simulink model "FKtest"  (Simulink 6.6)
settings: Solver=ode4  StartTime=0.0  StopTime=400  FixedStep=0.05  RelTol=1e-3
values from neighbouring files (symbols this model uses):
  vessel =     [input.mat]    (also in supply.mat)
undefined symbols (not defined in the file or in its folder): amp2
libraries: marine_gnc x21, simulink x5
(part 1 of 3)
settings Model: Creator=Thor  LastModifiedBy=Thor

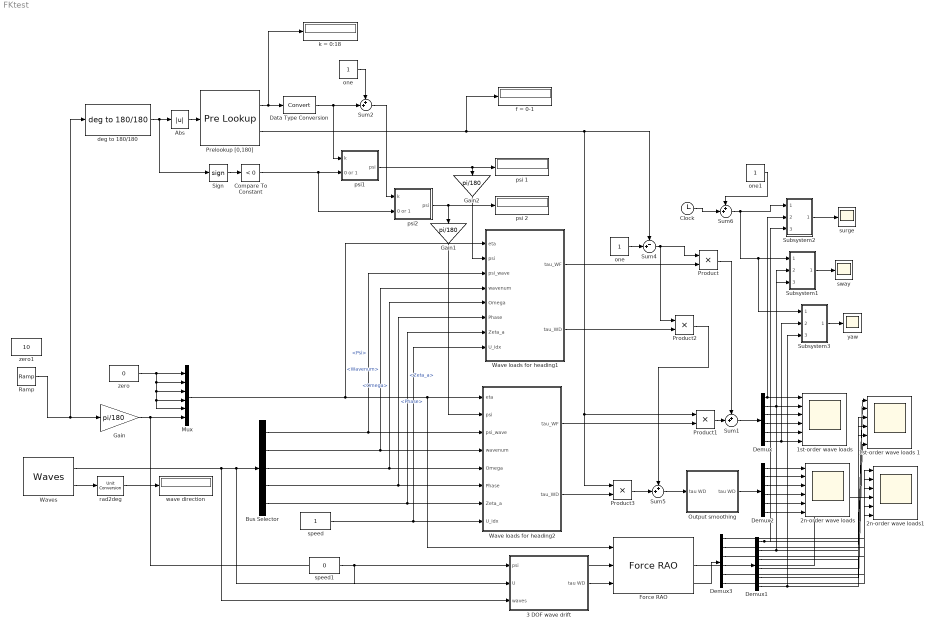
== system FKtest ==
  "1st-order wave loads " : Scope  NumInputPorts=6
      settings: TimeRange=100  YMin=-3e+006~-7e+006~-2e+007~-1e+007~-2e+008~-7.5e+007  YMax=2e+006~6e+006~1.5e+007~7.5e+006~2e+008~7.5e+007
  1st-order wave loads 1 : Scope  NumInputPorts=6
      settings: TimeRange=80  YMin=-4000000~-10000000~-20000000~-10000000~-400000000~-100000000  YMax=4000000~10000000~20000000~10000000~400000000~100000000  SaveName=ScopeData5
  2n-order wave loads : Scope  NumInputPorts=6
      settings: TimeRange=100  YMin=13750~80000~-1~-1~-1~270000  YMax=16250~160000~1~1~1~350000
  2n-order wave loads1 : Scope  NumInputPorts=6
      settings: TimeRange=100  YMin=11500~80000~-1~-1~-1~330000  YMax=17500~170000~1~1~1~420000  SaveName=ScopeData8
  3 DOF wave drift : Subsystem  AncestorBlock=hydro/Hydro Library/3 DOF wave drift  mask(Veres WD){WD_Freq=vessel.driftfrc.w, WD_Dir=vessel.headings, WD_Vel=vessel.velocities, WD_Amp=amp2, WD_add_omega_0=on, WD_add_omega_inf=on, RAO_yaw_quantization_flag=on, RAO_yaw_quant=5*pi/180, RAO_yaw_back=1.2*pi/180, RAO_speed_backlash_flag=on, RAO_speed_back=1, RAO_smoothing_flag=on, RAO_smoothing_T=5}
      mask prompts: WD_Freq "Vector of frequencies WD_Freq (rad/s)"; WD_Dir "Vector of directions WD_Dir (rad)"; WD_Vel "Vector of velocities WD_Vel (m/s)"; WD_Amp "3DOF Cell array with tables of Amplitudes WD_Amp"; WD_add_omega_0 "Add asymptotic WD values for omega = 0"; WD_add_omega_inf "Add asymptotic WD values for omega = inf"; RAO_yaw_quantization_flag "LF estimator for yaw angle table lookup (backlash and quantization)"; RAO_yaw_quant "LF yaw angle quantization interval [rad]"; RAO_yaw_back "LF yaw angle backlash width [rad] (typically 1/4 of the quantization interval)"; RAO_speed_backlash_flag "Speed lookup backlash (avoid rapid speed data switching)"; RAO_speed_back "Speed backlash widht [m/s]"; RAO_smoothing_flag "Filter wave drift forces to avoid steps due to table lookups"; RAO_smoothing_T "Time constant for wave drift force filter [s]"
      mask help:
      | Calculate the 6 degrees-of-freedom (DOF) 2nd order mean wave drift forces tau_WD for a vessel from its wave drift transfer functions (WDTFs) and a sea state defined by a set of harmonic waves. The block takes the "Waves" bus from the MSS Waves block as input, as well as the vessel low-frequency (LF) motion in terms of the yaw angle psi_LF and the mean surge velocity U.
      | The WDTFs are defined in terms of a vector of frequencies (WD_Freq), a vector of directions (WD_Dir), a vector of velocities (WD_Vel), and a 3DOF cell array of 3D matrices with amplitudes (WD_Amp), which are all input in the block mask. The first dimension of the 3D matrices corresponds to the frequencies, the second to the directions, and the third to the velocities, such that e.g. the amplitude amp in sway (DOF #2) for frequency number n_f, direction number n_d and velocity number n_v can be found from a = WD_Amp{2}(n_f, n_d, n_v). See help for details.
      |
      | Copyright (C) NTNU 2005
      |
      | Author: Oyvind N. Smogeli, 2005-05-11
      mask init:
      | % Add a second velocity if only one is given in order to avoid run-time errors in the table lookup blocks
      | if length(WD_Vel) == 1
      | 
      | 	if WD_Vel == 0 % Add a second identical data set for V = 5 m/s
      | 		WD_Vel(2) = 5;
      | 	else % Add a second identical data set for V = 0 m/s
      | 		WD_Vel = [0 WD_Vel];
      | 	end
      | 
      | 	for dofno = 1:3
      | 		WD_Amp{dofno}(:,:,2) = WD_Amp{dofno}(:,:,1);
      | 	end
      | 
      | end
      | 
      | if WD_add_omega_0 > 0
      | 	
      | 	if min(WD_Freq) > 0
      | 				
      | 		WD_Freq = [0 WD_Freq];
      | 		
      | 		for dofno = 1:3
      | 			WD_Amp{dofno} = [WD_Amp{dofno}(1,:,:); WD_Amp{dofno}];
      | 		end
      | 	
      | 	end
      | 	
      | end
      | 
      | maxfreq = 100;
      | nfreq = length(WD_Freq);
      | if WD_add_omega_inf > 0
      | 
      | 	if max(WD_Freq) < maxfreq
      | 			
      | 		newfreq = 2*max(WD_Freq) - WD_Freq(nfreq-1);
      | 		
      | 		WD_Freq = [WD_Freq newfreq maxfreq];
      | 		
      | 		for dofno = 1:3
      | 			WD_Amp{dofno} = [WD_Amp{dofno} ; WD_Amp{dofno}(nfreq,:,:) ; WD_Amp{dofno}(nfreq,:,:)];
      | 		end
      | 		
      | 	end
      | 
      | end
      mask Help:
      | <b>Part of the Marine Systems Simulator: MSS</b><br>
      | <br>
      | Calculate the 6 degrees-of-freedom (DOF) 2nd order mean wave drift forces tau_WD
      | for a vessel from its wave drift transfer functions (WDTFs) and a sea state
      | defined by a set of harmonic waves. The block takes the &quot;Waves&quot; bus from the MSS
      | Waves block as input, as well as the vessel low-frequency (LF) motion in terms
      | of the yaw angle psi_LF and the mean surge velocity U.<p>
      | The WDTFs are defined in terms of a vector of frequencies (WD_Freq), a vector of directions (WD_Dir), a vector of velocities (WD_Vel), and a 3DOF cell array of 3D matrices with amplitudes (WD_Amp), which are all input in the block mask. The first dimension of the 3D matrices corresponds to the frequencies, the second to the directions, and the third to the velocities, such that e.g. the amplitude amp in sway (DOF #2) for frequency number n_f, direction number n_d and velocity number n_v can be found from a = WD_Amp{2}(n_f, n_d, n_v).
      | See help for details.</p>
      | <p><b>Inputs:</b></p>
      | <p>Waves:&nbsp;&nbsp;&nbsp;&nbsp;&nbsp;&nbsp;&nbsp;&nbsp;&nbsp;&nbsp;&nbsp; Bus
      | containing the following signals<br>
      | &nbsp;&nbsp;&nbsp; Zeta_a:&nbsp;&nbsp;&nbsp;&nbsp;&nbsp;&nbsp;&nbsp; Vector of harmonic wave amplitudes [m]<br>
      | &nbsp;&nbsp;&nbsp; Omega:&nbsp;&nbsp;&nbsp;&nbsp;&nbsp;&nbsp; Vector of harmonic wave frequencies [rad/s]<br>
      | &nbsp;&nbsp;&nbsp; Phase:&nbsp;&nbsp;&nbsp;&nbsp;&nbsp;&nbsp;&nbsp;&nbsp; Vector of harmonic wave phases (random) [rad]<br>
      | &nbsp;&nbsp;&nbsp; Wavenum:&nbsp;&nbsp;&nbsp; Vector of harmonic wave numbers [1/m]<br>
      | &nbsp;&nbsp;&nbsp; Psi:&nbsp;&nbsp;&nbsp;&nbsp;&nbsp;&nbsp;&nbsp;&nbsp;&nbsp;&nbsp;&nbsp;&nbsp;&nbsp; Vector of harmonic wave directions [rad]</p>
      | <p>psi_LF:&nbsp;&nbsp;&nbsp;&nbsp;&nbsp;&nbsp;&nbsp;&nbsp;&nbsp;&nbsp;&nbsp;
      | Low-frequency vessel heading (Euler angle) [rad]</p>
      | <p>U&nbsp;&nbsp;&nbsp; :&nbsp;&nbsp;&nbsp;&nbsp;&nbsp;&nbsp;&nbsp;&nbsp;&nbsp;&nbsp;&nbsp;&nbsp;&nbsp;&nbsp;
      | Vessel low-frequency surge speed&nbsp; [m/s]</p>
      | <p><b>Outputs:</b></p>
      | <p>tau_WD:&nbsp;&nbsp;&nbsp;&nbsp;&nbsp;&nbsp;&nbsp;&nbsp;&nbsp; Generalized
      | 6DOF h-frame force vector [X (N), Y (N), Z (N), K (Nm), M (Nm), N (Nm)]</p>
      | <p><b>Model validity:</b></p>
      | <p>The validity of the block is dependent on the validity of the given
      | WD data set.</p>
      | <p>A proper WDTF to be used with this block should contain at least 1 velocity, 5
      | directions (e.g. 0, 45, 90, 135 and 180 degrees) and 10-20 frequencies, for all
      | 3 DOF (surge, sway, and yaw).</p>
      | <p>The block performs linear interpolation in frequencies and directions, and
      | uses the data set for the velocity closest to the input velocity (i.e. 'nearest'
      | interpolation in velocity). If the block recieves an input wave frequency or relative
      | wave direction outside the span of the data vectors WD_Freq or WD_Dir
      | respectively, the simulation stops and an error is returned. This means that a well-defined
      | WDTF must contain data for both 0 and 180 degrees, and for frequencies covering
      | the desired range of wave frequencies. If desired, asymptotic values can be
      | automatically added for zero and infinity frequency to avoid runtime errors if
      | the wave freqeuncy exceeds the values in WD_Freq (see checkboxes in the mask). </p>
      | <p>IMPORTANT NOTE: The theory upon which this block is based is in reality only
      | valid when the vessel low-frequency (h-frame) motion is a constant surge
      | velocity only, and the vessel is performing wave-frequency oscillations about
      | the steadily translating h-frame.This means that the outputs from the block when
      | manoeuvering -- i.e. changing the surge velocity and/or yaw angle -- must be
      | interpreted with some care. A jump in the output must be expected when changing
      | between two velocity data sets, and frequency warping expected when changing the
      | yaw angle (due to interpolation in the phase). It is therefore recommended to
      | use backlash on the input velocity to avoid transient switching, and a quantized
      | yaw angle with backlash. The latter will lead to jump in the ouput when the yaw
      | angle changes from one quantizied value to another, but will give better results
      | when keeping within one quantizer interval. The quantized yaw angle with
      | backlash and velocity with backlash are available as options via checkboxes in
      | the mask. If either of these are activated, proper values for the yaw
      | quantization interval, yaw backlash width, and the the speed backlash width
      | respectively must be set. Typical values could be a yaw quantization interval of
      | 5 degrees, yaw backlash width of 1/4-1/5 of the quantization interval, and speed
      | backlash width of 1 m/s. To avoid the most rapid transients when switching
      | between data sets, output smoothing is available as an option in the mask. If
      | this is enabled, the output during a transient is filtered by a 2nd order
      | transfer function with damping ratio 1 and eigenfrequency 1.5/T, where T is the
      | time constant specified in the mask.</p>
      | <p><b>Example mask input:</b></p><p>
      | As an example, the format of the mask input for 2 velocities, 3 directions and 5
      | frequencies is as follows:<p>WD_Freq = [f1 f2 f3 f4 f5]<br>
      | WD_Dir = [d1 d2 d3]<br>
      | WD_Vel = [v1 v2]<p>Surge:<br>
      | WD_Amp{1}(:,:,1)&nbsp; = [a1_111 a1_121 a1_131; a1_211 a1_221 a1_231; a1_311
      | a1_321 a1_331; a1_411 a1_421 a1_431; a1_511 a1_521 a1_531]<br>
      | WD_Amp{1}(:,:,2)&nbsp; = [a1_112 a1_122 a1_132; a1_212 a1_222 a1_232; a1_312
      | a1_322 a1_332; a1_412 a1_422 a1_432; a1_512 a1_522 a1_532]<br>
      | &nbsp;<p>Sway:<br>
      | WD_Amp{2}(:,:,1)&nbsp; = [a2_111 a2_121 a2_131; a2_211 a2_221 a2_231; a2_311
      | a2_321 a2_331; a2_411 a2_421 a2_431; a2_511 a2_521 a2_531]<br>
      | WD_Amp{2}(:,:,2)&nbsp; = [a2_112 a2_122 a2_132; a2_212 a2_222 a2_232; a2_312
      | a2_322 a2_332; a2_412 a2_422 a2_432; a2_512 a2_522 a2_532]<p>Yaw:<br>
      | WD_Amp{3}(:,:,1)&nbsp; = [a6_111 a6_121 a6_131; a6_211 a6_221 a6_231; a6_311
      | a6_321 a6_331; a6_411 a6_421 a6_431; a6_511 a6_521 a6_531]<br>
      | WD_Amp{3}(:,:,2)&nbsp; = [a6_112 a6_122 a6_132; a6_212 a6_222 a6_232; a6_312
      | a6_322 a6_332; a6_412 a6_422 a6_432; a6_512 a6_522 a6_532]<p>where now for example the
      | amplitude in sway (DOF 2) for frequency f5, direction d3 and velocity
      | v1 are given by WD_Amp{2}(5,3,1) = a2_531.<p>
      | <b>Copyright (C) NTNU 2005</b></p>
      | <p><b>Author:</b> Oyvind N. Smogeli, 2005-05-11</p>
  Abs : Abs  SaturateOnIntegerOverflow=on
  Bus Selector : BusSelector  OutputSignals=Psi,Wavenum,Omega,Phase,Zeta_a
  Clock : Clock
      settings: Decimation=10
  Compare To Constant : simulink/Logic and Bit Operations/Compare To Constant  SystemSampleTime=-1  relop=<  const=0  LogicOutDataTypeMode=uint8  ZeroCross=off
  Data Type Conversion : DataTypeConversion  OutDataTypeMode=double
  Demux{,1..3} (4 alike) : Demux  Outputs=6
  Force RAO : marine_gnc/Models/Environmental Loads/Force RAO  SystemSampleTime=-1  RAO_Freq=vessel.forceRAO.w  RAO_Dir=vessel.headings  RAO_Vel=vessel.velocities  RAO_Amp=amp  RAO_Phase=phase  RAO_add_omega_0=on  RAO_add_omega_inf=on  RAO_yaw_quantization_flag=on  RAO_yaw_quant=10*pi/180  RAO_yaw_back=2.5*pi/180  RAO_speed_backlash_flag=off  RAO_speed_back=1  RAO_smoothing_flag=on
  Gain : Gain  Gain=pi/180
  Gain1 : Gain  Orientation=down  Gain=pi/180
  Gain2 : Gain  Orientation=down  Gain=pi/180
  Mux : Mux  Inputs=6
  Output smoothing : Subsystem
  Prelookup [0,180] : PreLookup  BreakpointsData=[0:10:180]  IndexSearchMethod=Evenly spaced points  BeginIndexSearchUsingPreviousIndexResult=on
  Product{,1..3} (4 alike) : Product  RndMeth=Zero
  Ramp : simulink/Sources/Ramp  SystemSampleTime=-1  slope=1  start=0  X0=0
  Sign : Signum
  Subsystem1 : Subsystem
  Subsystem2 : Subsystem
  Subsystem3 : Subsystem
  Sum{1..2,5..6} (4 alike) : Sum  Inputs=++|
  Sum4 : Sum  Inputs=-+|
  Wave loads for heading1 : Subsystem  AncestorBlock=marine_gnc/Models/Environmental Loads/Force RAO  mask(Force RAO){ForceRAO_Freq=vessel.forceRAO.w, WD_Freq=vessel.driftfrc.w, RAO_Dir=vessel.headings, RAO_Vel=vessel.velocities, ForceRAO_Amp=vessel.forceRAO.amp, ForceRAO_Phase=vessel.forceRAO.phase, WD_Amp=vessel.driftfrc.amp, RAO_add_omega_0=on, RAO_add_omega_inf=on, RAO_speed_backlash_flag=off, RAO_speed_back=1}
      mask prompts: ForceRAO_Freq "Vector of frequencies ForceRAO_Freq (rad/s)"; WD_Freq "Vector of frequencies WD_Freq (rad/s)"; RAO_Dir "Vector of directions RAO_Dir (rad)"; RAO_Vel "Vector of velocities RAO_Vel (m/s)"; ForceRAO_Amp "6DOF Cell array with tables of Amplitudes ForceRAO_Amp"; ForceRAO_Phase "6DOF Cell array with tables of Phases ForceRAO_Phase (rad)"; WD_Amp "6DOF Cell array with tables of Amplitudes WD_Amp"; RAO_add_omega_0 "Add asymptotic RAO values for omega = 0"; RAO_add_omega_inf "Add asymptotic RAO values for omega = inf"; RAO_speed_backlash_flag "Speed lookup backlash (avoid rapid speed data switching)"; RAO_speed_back "Speed backlash widht [m/s]"
      mask help:
      | Calculate the 6 degrees-of-freedom (DOF) wave-frequency excitation forces Tau_WF for a vessel from its Force Response Amplitude Operators (Force RAOs) and a sea state defined by a set of harmonic waves. The block takes the "Waves" bus from the MSS Waves block as input, as well as the vessel low-frequency (LF) motion in terms of the generalized position vector eta_LF and mean surge velocity U. See help for details.
      |
      | Copyright (C) NTNU 2005
      | Author: Oyvind N. Smogeli, 2005-05-03
      mask init:
      | % Add RAO values for zero frequency: use values for lowest given frequency
      | if RAO_add_omega_0 > 0
      | 	
      | 	if min(ForceRAO_Freq) > 0
      | 				
      | 		ForceRAO_Freq = [0 ForceRAO_Freq];
      | 		for dofno = 1:6
      | 			ForceRAO_Amp{dofno}   = [ForceRAO_Amp{dofno}(1,:,:);   ForceRAO_Amp{dofno}];
      | 			ForceRAO_Phase{dofno} = [ForceRAO_Phase{dofno}(1,:,:); ForceRAO_Phase{dofno}];
      |         end
      | 
      |     end
      |     
      | 	if min(WD_Freq) > 0
      |         
      | 		WD_Freq = [0 WD_Freq];
      | 		for dofno = 1:3
      | 			WD_Amp{dofno} = [WD_Amp{dofno}(1,:,:); WD_Amp{dofno}];
      | 		end        
      |         
      | 	end
      | 	
      | end
      | 
      | % Add RAO values for high frequency: use values for highest given frequency
      | maxfreq = 100;
      | if RAO_add_omega_inf > 0
      | 
      | 	if max(ForceRAO_Freq) < maxfreq
      | 			
      | 		newfreq = 2*max(ForceRAO_Freq) - ForceRAO_Freq(length(ForceRAO_Freq)-1);
      | 		
      | 		ForceRAO_Freq = [ForceRAO_Freq newfreq maxfreq];
      | 		for dofno = 1:6
      | 			ForceRAO_Amp{dofno}   = [ForceRAO_Amp{dofno};   zeros(2, length(RAO_Dir), 10)];
      | 			ForceRAO_Phase{dofno} = [ForceRAO_Phase{dofno}; zeros(2, length(RAO_Dir), 10)];
      | 		end
      | 		
      |     end
      | 
      | 	if max(WD_Freq) < maxfreq
      | 			
      | 		newfreq = 2*max(WD_Freq) - WD_Freq(length(WD_Freq)-1);
      | 		
      | 		WD_Freq = [WD_Freq newfreq maxfreq];
      | 		for dofno = 1:3
      | 			WD_Amp{dofno} = [WD_Amp{dofno}; zeros(2, length(RAO_Dir), 10)];
      | 		end
      | 		
      |     end
      |     
      | end
      mask Help:
      | <b>Part of the Marine Systems Simulator: MSS</b><br>
      | <br>
      | Calculate the 6 degrees-of-freedom (DOF) wave-frequency excitation forces Tau_WF
      | for a vessel from its Force Response Amplitude Operators (Force RAOs) and a sea
      | state defined by a set of harmonic waves. The block takes the &quot;Waves&quot; bus from
      | the MSS Waves block as input, as well as the vessel low-frequency (LF) motion in
      | terms of the generalized position vector eta_LF and mean surge velocity U.<p>The Force RAOs are defined in terms of a
      | vector of frequencies (RAO_Freq), a vector of directions (RAO_Dir), a vector of
      | velocities (RAO_Dir), a 6DOF cell array of 3D matrices with amplitudes
      | (RAO_Amp), and a 6DOF cell array of 3D matrices with phases (RAO_Phase), which
      | are all input in the block mask. The first dimension of the 3D matrices
      | corresponds to the frequencies, the second to the directions, and the third to
      | the velocities, such that e.g. the amplitude amp in heave (DOF #3) for frequency
      | number n_f, direction number n_d and velocity number n_v can be found from a =
      | RAO_Amp{3}(n_f, n_d, n_v).</p>
      | <p><b>Inputs:</b></p>
      | <p>Waves:&nbsp;&nbsp;&nbsp;&nbsp;&nbsp;&nbsp;&nbsp;&nbsp;&nbsp;&nbsp;&nbsp; Bus
      | containing the following signals<br>
      | &nbsp;&nbsp;&nbsp; Zeta_a:&nbsp;&nbsp;&nbsp;&nbsp;&nbsp;&nbsp;&nbsp; Vector of harmonic wave amplitudes [m]<br>
      | &nbsp;&nbsp;&nbsp; Omega:&nbsp;&nbsp;&nbsp;&nbsp;&nbsp;&nbsp; Vector of harmonic wave frequencies [rad/s]<br>
      | &nbsp;&nbsp;&nbsp; Phase:&nbsp;&nbsp;&nbsp;&nbsp;&nbsp;&nbsp;&nbsp;&nbsp; Vector of harmonic wave phases (random) [rad]<br>
      | &nbsp;&nbsp;&nbsp; Wavenum:&nbsp;&nbsp;&nbsp; Vector of harmonic wave numbers [1/m]<br>
      | &nbsp;&nbsp;&nbsp; Psi:&nbsp;&nbsp;&nbsp;&nbsp;&nbsp;&nbsp;&nbsp;&nbsp;&nbsp;&nbsp;&nbsp;&nbsp;&nbsp; Vector of harmonic wave directions [rad]</p>
      | <p>eta_LF:&nbsp;&nbsp;&nbsp;&nbsp;&nbsp;&nbsp;&nbsp;&nbsp;&nbsp;&nbsp;&nbsp;
      | Generalized 6DOF n-frame low-frequency position vector [x (m), y (m), z (m),
      | theta (rad), phi (rad), psi (rad)]<br>
      | U:&nbsp;&nbsp;&nbsp;&nbsp;&nbsp;&nbsp;&nbsp;&nbsp;&nbsp;&nbsp;&nbsp;&nbsp;&nbsp;&nbsp;&nbsp;&nbsp;&nbsp;&nbsp;&nbsp;
      | Low-frequency (mean) surge velocity&nbsp; [m/s]</p>
      | <p><b>Outputs:</b></p>
      | <p>tau_WF:&nbsp;&nbsp;&nbsp;&nbsp;&nbsp;&nbsp;&nbsp;&nbsp;&nbsp; Generalized
      | 6DOF h-frame force vector [X (N), Y (N), Z (N), K (Nm), M (Nm), N (Nm)]</p>
      | <p><b>Model validity:</b></p>
      | <p>The validity of the block is dependent on the validity of the given
      | RAO data set.</p>
      | <p>A proper RAO to be used with this block should contain at least 1 velocity, 5
      | directions (e.g. 0, 45, 90, 135 and 180 degrees) and 10-20 frequencies, for all
      | 6 DOF (surge, sway, heave, roll, pitch, yaw).</p>
      | <p>The block performs linear interpolation in frequencies and directions, and
      | uses the data set for the velocity closest to the input velocity (i.e. 'nearest'
      | interpolation in velocity). If the block recieves an input wave frequency or relative
      | wave direction outside the span of the data vectors RAO_Freq or RAO_Dir
      | respectively, the simulation stops and an error is returned. This means that a well-defined
      | RAO must contain data for both 0 and 180 degrees, and for frequencies covering
      | the desired range of wave frequencies. If desired, asymptotic values can be
      | automatically added for zero and infinity frequency to avoid runtime errors if
      | the wave freqeuncy exceeds the values in RAO_Freq (see checkboxes in the mask). </p>
      | <p>IMPORTANT NOTE: The RAO theory upon which this block is based is in reality
      | only valid when the vessel low-frequency (h-frame) motion is a constant surge
      | velocity only, and the vessel is performing wave-frequency oscillations about
      | the steadily translating h-frame.This means that the outputs from the block when
      | manoeuvering -- i.e. changing the surge velocity and/or yaw angle -- must be
      | interpreted with some care. A jump in the output must be expected when changing
      | between two velocity data sets, and frequency warping expected when changing the
      | yaw angle (due to interpolation in the phase). It is therefore recommended to
      | use backlash on the input velocity to avoid transient switching, and a quantized
      | yaw angle with backlash. The latter will lead to jump in the ouput when the yaw
      | angle changes from one quantized value to another, but will give better results
      | when keeping within one quantizer interval. The quantized yaw angle with
      | backlash and velocity with backlash are available as options via checkboxes in
      | the mask. If either of these are activated, proper values for the yaw
      | quantization interval, yaw backlash width, and the the speed backlash width
      | respectively must be set. Typical values could be a yaw quantization interval of
      | 5 degrees, yaw backlash width of 1/4-1/5 of the quantization interval, and speed
      | backlash width of 1 m/s. To avoid the most rapid transients when switching
      | between data sets, output smoothing is available as an option in the mask. If
      | this is enabled, the output during a transent is rate limited according to the
      | fastest recorded signal rate during normal operation.</p>
      | <p><b>Example mask input:</b></p><p>
      | As an example, the format of the mask input for 2 velocities, 3 directions and 5
      | frequencies is as follows:<p>RAO_Freq = [f1 f2 f3 f4 f5]<br>
      | RAO_Dir = [d1 d2 d3]<br>
      | RAO_Vel = [v1 v2]<p>Surge:<br>
      | RAO_Amp{1}(:,:,1)&nbsp; = [a1_111 a1_121 a1_131; a1_211 a1_221 a1_231; a1_311
      | a1_321 a1_331; a1_411 a1_421 a1_431; a1_511 a1_521 a1_531]<br>
      | RAO_Amp{1}(:,:,2)&nbsp; = [a1_112 a1_122 a1_132; a1_212 a1_222 a1_232; a1_312
      | a1_322 a1_332; a1_412 a1_422 a1_432; a1_512 a1_522 a1_532]<br>
      | RAO_Phase{1}(:,:,1) = [p1_111 p1_121 p1_131; p1_211 p1_221 p1_231; p1_311 p1_321
      | p1_331; p1_411 p1_421 p1_431; p1_511 p1_521 p1_531]<br>
      | RAO_Phase{1}(:,:,2) = [p1_112 p1_122 p1_132; p1_212 p1_222 p1_232; p1_312 p1_322
      | p1_332; p1_412 p1_422 p1_432; p1_512 p1_522 p1_532]<p>Sway:<br>
      | RAO_Amp{2}(:,:,1)&nbsp; = [a2_111 a2_121 a2_131; a2_211 a2_221 a2_231; a2_311
      | a2_321 a2_331; a2_411 a2_421 a2_431; a2_511 a2_521 a2_531]<br>
      | RAO_Amp{2}(:,:,2)&nbsp; = [a2_112 a2_122 a2_132; a2_212 a2_222 a2_232; a2_312
      | a2_322 a2_332; a2_412 a2_422 a2_432; a2_512 a2_522 a2_532]<br>
      | RAO_Phase{2}(:,:,1) = [p2_111 p2_121 p2_131; p2_211 p2_221 p2_231; p2_311 p2_321
      | p2_331; p2_411 p2_421 p2_431; p2_511 p2_521 p2_531]<br>
      | RAO_Phase{2}(:,:,2) = [p2_112 p2_122 p2_132; p2_212 p2_222 p2_232; p2_312 p2_322
      | p2_332; p2_412 p2_422 p2_432; p2_512 p2_522 p2_532]<p>...<p>Yaw:<br>
      | RAO_Amp{6}(:,:,1)&nbsp; = [a6_111 a6_121 a6_131; a6_211 a6_221 a6_231; a6_311
      | a6_321 a6_331; a6_411 a6_421 a6_431; a6_511 a6_521 a6_531]<br>
      | RAO_Amp{6}(:,:,2)&nbsp; = [a6_112 a6_122 a6_132; a6_212 a6_222 a6_232; a6_312
      | a6_322 a6_332; a6_412 a6_422 a6_432; a6_512 a6_522 a6_532]<br>
      | RAO_Phase{6}(:,:,1) = [p6_111 p6_121 p6_131; p6_211 p6_221 p6_231; p6_311 p6_321
      | p6_331; p6_411 p6_421 p6_431; p6_511 p6_521 p6_531]<br>
      | RAO_Phase{6}(:,:,2) = [p6_112 p6_122 p6_132; p6_212 p6_222 p6_232; p6_312 p6_322
      | p6_332; p6_412 p6_422 p6_432; p6_512 p6_522 p6_532]<p>where now for example the
      | amplitude and phase in sway (DOF 2) for frequency f5, direction d3 and velocity
      | v1 are given by RAO_Amp{2}(5,3,1) = a2_531 and RAO_Phase{2}(5,3,1) = p2_531.<p>
      | <b>Copyright (C) NTNU 2005</b></p>
      | <p><b>Author:</b> Oyvind N. Smogeli, 2005-05-03</p>
  Wave loads for heading2 : Subsystem  AncestorBlock=marine_gnc/Models/Environmental Loads/Force RAO  mask(Force RAO){ForceRAO_Freq=vessel.forceRAO.w, WD_Freq=vessel.driftfrc.w, RAO_Dir=vessel.headings, RAO_Vel=vessel.velocities, ForceRAO_Amp=vessel.forceRAO.amp, ForceRAO_Phase=vessel.forceRAO.phase, WD_Amp=vessel.driftfrc.amp, RAO_add_omega_0=on, RAO_add_omega_inf=on, RAO_speed_backlash_flag=off, RAO_speed_back=1}
      mask prompts: ForceRAO_Freq "Vector of frequencies ForceRAO_Freq (rad/s)"; WD_Freq "Vector of frequencies WD_Freq (rad/s)"; RAO_Dir "Vector of directions RAO_Dir (rad)"; RAO_Vel "Vector of velocities RAO_Vel (m/s)"; ForceRAO_Amp "6DOF Cell array with tables of Amplitudes ForceRAO_Amp"; ForceRAO_Phase "6DOF Cell array with tables of Phases ForceRAO_Phase (rad)"; WD_Amp "6DOF Cell array with tables of Amplitudes WD_Amp"; RAO_add_omega_0 "Add asymptotic RAO values for omega = 0"; RAO_add_omega_inf "Add asymptotic RAO values for omega = inf"; RAO_speed_backlash_flag "Speed lookup backlash (avoid rapid speed data switching)"; RAO_speed_back "Speed backlash widht [m/s]"
      mask help:
      | Calculate the 6 degrees-of-freedom (DOF) wave-frequency excitation forces Tau_WF for a vessel from its Force Response Amplitude Operators (Force RAOs) and a sea state defined by a set of harmonic waves. The block takes the "Waves" bus from the MSS Waves block as input, as well as the vessel low-frequency (LF) motion in terms of the generalized position vector eta_LF and mean surge velocity U. See help for details.
      |
      | Copyright (C) NTNU 2005
      | Author: Oyvind N. Smogeli, 2005-05-03
      mask init: same as FKtest/Wave loads for heading1
      mask Help:
      | <b>Part of the Marine Systems Simulator: MSS</b><br>
      | <br>
      | Calculate the 6 degrees-of-freedom (DOF) wave-frequency excitation forces Tau_WF
      | for a vessel from its Force Response Amplitude Operators (Force RAOs) and a sea
      | state defined by a set of harmonic waves. The block takes the &quot;Waves&quot; bus from
      | the MSS Waves block as input, as well as the vessel low-frequency (LF) motion in
      | terms of the generalized position vector eta_LF and mean surge velocity U.<p>The Force RAOs are defined in terms of a
      | vector of frequencies (RAO_Freq), a vector of directions (RAO_Dir), a vector of
      | velocities (RAO_Dir), a 6DOF cell array of 3D matrices with amplitudes
      | (RAO_Amp), and a 6DOF cell array of 3D matrices with phases (RAO_Phase), which
      | are all input in the block mask. The first dimension of the 3D matrices
      | corresponds to the frequencies, the second to the directions, and the third to
      | the velocities, such that e.g. the amplitude amp in heave (DOF #3) for frequency
      | number n_f, direction number n_d and velocity number n_v can be found from a =
      | RAO_Amp{3}(n_f, n_d, n_v).</p>
      | <p><b>Inputs:</b></p>
      | <p>Waves:&nbsp;&nbsp;&nbsp;&nbsp;&nbsp;&nbsp;&nbsp;&nbsp;&nbsp;&nbsp;&nbsp; Bus
      | containing the following signals<br>
      | &nbsp;&nbsp;&nbsp; Zeta_a:&nbsp;&nbsp;&nbsp;&nbsp;&nbsp;&nbsp;&nbsp; Vector of harmonic wave amplitudes [m]<br>
      | &nbsp;&nbsp;&nbsp; Omega:&nbsp;&nbsp;&nbsp;&nbsp;&nbsp;&nbsp; Vector of harmonic wave frequencies [rad/s]<br>
      | &nbsp;&nbsp;&nbsp; Phase:&nbsp;&nbsp;&nbsp;&nbsp;&nbsp;&nbsp;&nbsp;&nbsp; Vector of harmonic wave phases (random) [rad]<br>
      | &nbsp;&nbsp;&nbsp; Wavenum:&nbsp;&nbsp;&nbsp; Vector of harmonic wave numbers [1/m]<br>
      | &nbsp;&nbsp;&nbsp; Psi:&nbsp;&nbsp;&nbsp;&nbsp;&nbsp;&nbsp;&nbsp;&nbsp;&nbsp;&nbsp;&nbsp;&nbsp;&nbsp; Vector of harmonic wave directions [rad]</p>
      | <p>eta_LF:&nbsp;&nbsp;&nbsp;&nbsp;&nbsp;&nbsp;&nbsp;&nbsp;&nbsp;&nbsp;&nbsp;
      | Generalized 6DOF n-frame low-frequency position vector [x (m), y (m), z (m),
      | theta (rad), phi (rad), psi (rad)]<br>
      | U:&nbsp;&nbsp;&nbsp;&nbsp;&nbsp;&nbsp;&nbsp;&nbsp;&nbsp;&nbsp;&nbsp;&nbsp;&nbsp;&nbsp;&nbsp;&nbsp;&nbsp;&nbsp;&nbsp;
      | Low-frequency (mean) surge velocity&nbsp; [m/s]</p>
      | <p><b>Outputs:</b></p>
      | <p>tau_WF:&nbsp;&nbsp;&nbsp;&nbsp;&nbsp;&nbsp;&nbsp;&nbsp;&nbsp; Generalized
      | 6DOF h-frame force vector [X (N), Y (N), Z (N), K (Nm), M (Nm), N (Nm)]</p>
      | <p><b>Model validity:</b></p>
      | <p>The validity of the block is dependent on the validity of the given
      | RAO data set.</p>
      | <p>A proper RAO to be used with this block should contain at least 1 velocity, 5
      | directions (e.g. 0, 45, 90, 135 and 180 degrees) and 10-20 frequencies, for all
      | 6 DOF (surge, sway, heave, roll, pitch, yaw).</p>
      | <p>The block performs linear interpolation in frequencies and directions, and
      | uses the data set for the velocity closest to the input velocity (i.e. 'nearest'
      | interpolation in velocity). If the block recieves an input wave frequency or relative
      | wave direction outside the span of the data vectors RAO_Freq or RAO_Dir
      | respectively, the simulation stops and an error is returned. This means that a well-defined
      | RAO must contain data for both 0 and 180 degrees, and for frequencies covering
      | the desired range of wave frequencies. If desired, asymptotic values can be
      | automatically added for zero and infinity frequency to avoid runtime errors if
      | the wave freqeuncy exceeds the values in RAO_Freq (see checkboxes in the mask). </p>
      | <p>IMPORTANT NOTE: The RAO theory upon which this block is based is in reality
      | only valid when the vessel low-frequency (h-frame) motion is a constant surge
      | velocity only, and the vessel is performing wave-frequency oscillations about
      | the steadily translating h-frame.This means that the outputs from the block when
      | manoeuvering -- i.e. changing the surge velocity and/or yaw angle -- must be
      | interpreted with some care. A jump in the output must be expected when changing
      | between two velocity data sets, and frequency warping expected when changing the
      | yaw angle (due to interpolation in the phase). It is therefore recommended to
      | use backlash on the input velocity to avoid transient switching, and a quantized
      | yaw angle with backlash. The latter will lead to jump in the ouput when the yaw
      | angle changes from one quantized value to another, but will give better results
      | when keeping within one quantizer interval. The quantized yaw angle with
      | backlash and velocity with backlash are available as options via checkboxes in
      | the mask. If either of these are activated, proper values for the yaw
      | quantization interval, yaw backlash width, and the the speed backlash width
      | respectively must be set. Typical values could be a yaw quantization interval of
      | 5 degrees, yaw backlash width of 1/4-1/5 of the quantization interval, and speed
      | backlash width of 1 m/s. To avoid the most rapid transients when switching
      | between data sets, output smoothing is available as an option in the mask. If
      | this is enabled, the output during a transent is rate limited according to the
      | fastest recorded signal rate during normal operation.</p>
      | <p><b>Example mask input:</b></p><p>
      | As an example, the format of the mask input for 2 velocities, 3 directions and 5
      | frequencies is as follows:<p>RAO_Freq = [f1 f2 f3 f4 f5]<br>
      | RAO_Dir = [d1 d2 d3]<br>
      | RAO_Vel = [v1 v2]<p>Surge:<br>
      | RAO_Amp{1}(:,:,1)&nbsp; = [a1_111 a1_121 a1_131; a1_211 a1_221 a1_231; a1_311
      | a1_321 a1_331; a1_411 a1_421 a1_431; a1_511 a1_521 a1_531]<br>
      | RAO_Amp{1}(:,:,2)&nbsp; = [a1_112 a1_122 a1_132; a1_212 a1_222 a1_232; a1_312
      | a1_322 a1_332; a1_412 a1_422 a1_432; a1_512 a1_522 a1_532]<br>
      | RAO_Phase{1}(:,:,1) = [p1_111 p1_121 p1_131; p1_211 p1_221 p1_231; p1_311 p1_321
      | p1_331; p1_411 p1_421 p1_431; p1_511 p1_521 p1_531]<br>
      | RAO_Phase{1}(:,:,2) = [p1_112 p1_122 p1_132; p1_212 p1_222 p1_232; p1_312 p1_322
      | p1_332; p1_412 p1_422 p1_432; p1_512 p1_522 p1_532]<p>Sway:<br>
      | RAO_Amp{2}(:,:,1)&nbsp; = [a2_111 a2_121 a2_131; a2_211 a2_221 a2_231; a2_311
      | a2_321 a2_331; a2_411 a2_421 a2_431; a2_511 a2_521 a2_531]<br>
      | RAO_Amp{2}(:,:,2)&nbsp; = [a2_112 a2_122 a2_132; a2_212 a2_222 a2_232; a2_312
      | a2_322 a2_332; a2_412 a2_422 a2_432; a2_512 a2_522 a2_532]<br>
      | RAO_Phase{2}(:,:,1) = [p2_111 p2_121 p2_131; p2_211 p2_221 p2_231; p2_311 p2_321
      | p2_331; p2_411 p2_421 p2_431; p2_511 p2_521 p2_531]<br>
      | RAO_Phase{2}(:,:,2) = [p2_112 p2_122 p2_132; p2_212 p2_222 p2_232; p2_312 p2_322
      | p2_332; p2_412 p2_422 p2_432; p2_512 p2_522 p2_532]<p>...<p>Yaw:<br>
      | RAO_Amp{6}(:,:,1)&nbsp; = [a6_111 a6_121 a6_131; a6_211 a6_221 a6_231; a6_311
      | a6_321 a6_331; a6_411 a6_421 a6_431; a6_511 a6_521 a6_531]<br>
      | RAO_Amp{6}(:,:,2)&nbsp; = [a6_112 a6_122 a6_132; a6_212 a6_222 a6_232; a6_312
      | a6_322 a6_332; a6_412 a6_422 a6_432; a6_512 a6_522 a6_532]<br>
      | RAO_Phase{6}(:,:,1) = [p6_111 p6_121 p6_131; p6_211 p6_221 p6_231; p6_311 p6_321
      | p6_331; p6_411 p6_421 p6_431; p6_511 p6_521 p6_531]<br>
      | RAO_Phase{6}(:,:,2) = [p6_112 p6_122 p6_132; p6_212 p6_222 p6_232; p6_312 p6_322
      | p6_332; p6_412 p6_422 p6_432; p6_512 p6_522 p6_532]<p>where now for example the
      | amplitude and phase in sway (DOF 2) for frequency f5, direction d3 and velocity
      | v1 are given by RAO_Amp{2}(5,3,1) = a2_531 and RAO_Phase{2}(5,3,1) = p2_531.<p>
      | <b>Copyright (C) NTNU 2005</b></p>
      | <p><b>Author:</b> Oyvind N. Smogeli, 2005-05-03</p>
  Waves : marine_gnc/Environment/Waves/Waves  SystemSampleTime=-1  spectrum_type=ITTC  disp_flag=off  plot_spectrum=off  plot_realization=off  hs=5  omega_peak=-1  psi_mean=0/(180/pi)  gamma=-1  spread=2  depth=inf  nfreq=20  ndir=10  energylim=0.005  freq_cutoff=3  dir_cutoff=0  rand_seed=0  rand_freq=on  rand_dir=on  Zeta_a=0  Omega=0  Phase=0  Wavenum=0  Psi=0
  deg to 180/180 : marine_gnc/Utilities/Math Operations/deg to 180//180  SystemSampleTime=-1
  f = 0-1 : Display
  k = 0:18 : Display
  one : Constant
  "one " : Constant
  one1 : Constant
  psi 1 : Display
  psi 2 : Display
  psi1 : Subsystem
  psi2 : Subsystem
  rad2deg : marine_gnc/Utilities/Math Operations/Unit Conversion  SystemSampleTime=-1  in=rad2deg
  speed : Constant
  speed1 : Constant  Value=0
  surge : Scope
      settings: YMin=-1.4e+006  YMax=900000  SaveName=ScopeData4
  sway : Scope
      settings: YMin=-350000  YMax=100000  SaveName=ScopeData6
  wave direction : Display
  yaw : Scope
      settings: YMin=-2.5e+006  YMax=500000  SaveName=ScopeData7
  zero : Constant  Value=0
  zero1 : Constant  Value=10
  wires:
  speed/1 -> Wave loads for heading1/8(U_idx), Wave loads for heading2/8(U_idx)
  Ramp/1 -> Gain/1, deg to 180/180/1
  Waves/2 -> rad2deg/1
  rad2deg/1 -> wave direction/1
  Demux/1 -> "1st-order wave loads "/1, Subsystem2/2(In2)
  Demux/2 -> "1st-order wave loads "/2, Subsystem1/2(In2)
  Demux/3 -> "1st-order wave loads "/3
  Demux/4 -> "1st-order wave loads "/4
  Demux/5 -> "1st-order wave loads "/5
  Demux/6 -> "1st-order wave loads "/6, Subsystem3/2(In2)
  Wave loads for heading2/1(tau_WF) -> Product1/2
  Demux2/1 -> 2n-order wave loads/1
  Demux2/2 -> 2n-order wave loads/2
  Demux2/3 -> 2n-order wave loads/3
  Demux2/4 -> 2n-order wave loads/4
  Demux2/5 -> 2n-order wave loads/5
  Demux2/6 -> 2n-order wave loads/6
  Wave loads for heading2/2(tau_WD) -> Product3/2
  Mux/1 -> Wave loads for heading1/1(eta), Wave loads for heading2/1(eta), Force RAO/1
  zero/1 -> Mux/1, Mux/2, Mux/3, Mux/4, Mux/5
  Bus Selector/1 -> Wave loads for heading1/3(psi_wave), Wave loads for heading2/3(psi_wave)  "<Psi>"
  Waves/1 -> Bus Selector/1, Force RAO/3, 3 DOF wave drift/3(waves)
  Bus Selector/2 -> Wave loads for heading1/4(wavenum), Wave loads for heading2/4(wavenum)  "<Wavenum>"
  Bus Selector/3 -> Wave loads for heading1/5(Omega), Wave loads for heading2/5(Omega)  "<Omega>"
  Bus Selector/4 -> Wave loads for heading1/6(Phase), Wave loads for heading2/6(Phase)  "<Phase>"
  Bus Selector/5 -> Wave loads for heading1/7(Zeta_a), Wave loads for heading2/7(Zeta_a)  "<Zeta_a>"
  Prelookup [0,180]/1 -> Data Type Conversion/1, k = 0:18/1
  one/1 -> Sum2/1
  Sum2/1 -> psi2/1(k)
  Gain/1 -> Mux/6, 3 DOF wave drift/1(psi)
  Sum1/1 -> Demux/1
  Wave loads for heading1/1(tau_WF) -> Product/2
  Product/1 -> Sum1/1
  Product1/1 -> Sum1/2
  "one "/1 -> Sum4/2
  Sum4/1 -> Product/1, Product2/1
  Wave loads for heading1/2(tau_WD) -> Product2/2
  Product3/1 -> Sum5/2
  Product2/1 -> Sum5/1
  Output smoothing/1("tau WD ") -> Demux2/1
  speed1/1 -> Force RAO/2, 3 DOF wave drift/2(U)
  Demux1/1 -> 1st-order wave loads 1/1, Subsystem2/3(In3)
  Demux1/2 -> 1st-order wave loads 1/2, Subsystem1/3(In3)
  Demux1/3 -> 1st-order wave loads 1/3
  Demux1/4 -> 1st-order wave loads 1/4
  Demux1/5 -> 1st-order wave loads 1/5
  Demux1/6 -> 1st-order wave loads 1/6, Subsystem3/3(In3)
  Force RAO/1 -> Demux1/1
  Subsystem2/1(Out1) -> surge/1
  one1/1 -> Sum6/1
  Clock/1 -> Sum6/2
  Sum6/1 -> Subsystem2/1(In1), Subsystem1/1(In1), Subsystem3/1(In1)
  Subsystem1/1(Out1) -> sway/1
  Subsystem3/1(Out1) -> yaw/1
  Demux3/1 -> 2n-order wave loads1/1
  Demux3/2 -> 2n-order wave loads1/2
  Demux3/3 -> 2n-order wave loads1/3
  Demux3/4 -> 2n-order wave loads1/4
  Demux3/5 -> 2n-order wave loads1/5
  Demux3/6 -> 2n-order wave loads1/6
  3 DOF wave drift/1(tau WD) -> Demux3/1
  Sum5/1 -> Output smoothing/1(tau WD)
  deg to 180/180/1 -> Abs/1, Sign/1
  Abs/1 -> Prelookup [0,180]/1
  Sign/1 -> Compare To Constant/1
  Compare To Constant/1 -> psi1/2(0 or 1), psi2/2(0 or 1)
  psi1/1(psi) -> psi 1/1, Gain2/1
  Prelookup [0,180]/2 -> Sum4/1, Product3/1, Product1/1, f = 0-1/1
  Data Type Conversion/1 -> Sum2/2, psi1/1(k)
  psi2/1(psi) -> psi 2/1, Gain1/1
  Gain1/1 -> Wave loads for heading2/2(psi)
  Gain2/1 -> Wave loads for heading1/2(psi)

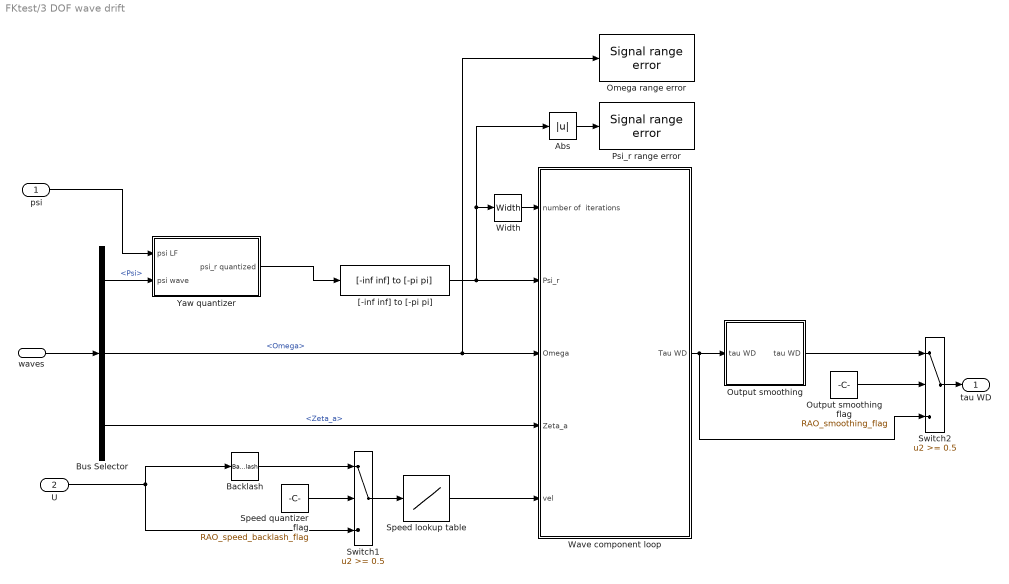
== system FKtest/3 DOF wave drift ==
  psi : Inport
  U : Inport  Port=2
  waves : Inport  Port=3
  Abs : Abs
  Backlash : Backlash  BacklashWidth=RAO_speed_back
  Bus Selector : BusSelector  OutputSignals=Psi,Omega,Zeta_a
  Omega range error : marine_gnc/Utilities/Simulation tools/Signal range error  SystemSampleTime=-1  Values=WD_Freq  message=Wave frequency outside range of Wavedrift table
  Output smoothing flag : Constant  Value=RAO_smoothing_flag
  Output smoothing : Subsystem
  Psi_r range error : marine_gnc/Utilities/Simulation tools/Signal range error  SystemSampleTime=-1  Values=WD_Dir  message=Relative wave direction outside range of Wavedrift table
  Speed lookup table : Lookup  InputValues=WD_Vel  OutputValues=WD_Vel  LookUpMeth=Use Input Nearest
  Speed quantizer flag : Constant  Value=RAO_speed_backlash_flag
  Switch1 : Switch  Threshold=0.5
  Switch2 : Switch  Threshold=0.5
  Wave component loop : Subsystem  TreatAsAtomicUnit=on
  Width : Width  DataType=int32
  Yaw quantizer : Subsystem  AncestorBlock=marine_gnc/Models/Environmental Loads/Utilities/Yaw quantizer  mask(Yaw quantizer){quant_flag=RAO_yaw_quantization_flag, quant=RAO_yaw_quant, back=RAO_yaw_back}
      mask prompts: quant_flag "Quantizer flag {0,1}"; quant "Quantizer interval [rad]"; back "Backlash width [rad]"
      mask help: Apply quantization and backlash to the yaw angle if desired, and calculate the wave direction relative to the vessel. If the quantizer flag is set to zero, the two outputs are equal.
  "[-inf inf] to [-pi pi]" : marine_gnc/Utilities/Math Operations/[-inf inf] to [-pi pi]  SystemSampleTime=-1
  tau WD : Outport
  wires:
  waves/1 -> Bus Selector/1
  Bus Selector/1 -> Yaw quantizer/2(psi wave)  "<Psi>"
  Bus Selector/2 -> Wave component loop/3(Omega), Omega range error/1  "<Omega>"
  Bus Selector/3 -> Wave component loop/4(Zeta_a)  "<Zeta_a>"
  Width/1 -> Wave component loop/1(number of  iterations)
  "[-inf inf] to [-pi pi]"/1 -> Wave component loop/2(Psi_r), Width/1, Abs/1
  Abs/1 -> Psi_r range error/1
  Speed lookup table/1 -> Wave component loop/5(vel)
  Switch1/1 -> Speed lookup table/1
  Backlash/1 -> Switch1/1
  Speed quantizer flag/1 -> Switch1/2
  U/1 -> Backlash/1, Switch1/3
  Yaw quantizer/1(psi_r quantized) -> "[-inf inf] to [-pi pi]"/1
  psi/1 -> Yaw quantizer/1(psi LF)
  Output smoothing flag/1 -> Switch2/2
  Switch2/1 -> tau WD/1
  Wave component loop/1(Tau WD) -> Switch2/3, Output smoothing/1(tau WD)
  Output smoothing/1("tau WD ") -> Switch2/1

== system FKtest/Output smoothing ==
  tau WD : Inport
  2nd order time constant 1 : marine_gnc/Utilities/Dynamics/2nd order time constant  SystemSampleTime=-1  T=5
  2nd order time constant 2 : marine_gnc/Utilities/Dynamics/2nd order time constant  SystemSampleTime=-1  T=5
  2nd order time constant 6 : marine_gnc/Utilities/Dynamics/2nd order time constant  SystemSampleTime=-1  T=5
  Demux : Demux  Outputs=6
  Mux : Mux  Inputs=6
  "tau WD " : Outport
  wires:
  Demux/1 -> 2nd order time constant 1/1
  Demux/2 -> 2nd order time constant 2/1
  Demux/3 -> Mux/3
  Demux/4 -> Mux/4
  Demux/5 -> Mux/5
  Demux/6 -> 2nd order time constant 6/1
  tau WD/1 -> Demux/1
  2nd order time constant 1/1 -> Mux/1
  2nd order time constant 2/1 -> Mux/2
  2nd order time constant 6/1 -> Mux/6
  Mux/1 -> "tau WD "/1

== system FKtest/Subsystem1 ==
  In1 : Inport
  In2 : Inport  Port=2
  In3 : Inport  Port=3
  Mux2 : Mux  Inputs=2
  Subsystem : Subsystem
  Subsystem1 : Subsystem
  Out1 : Outport
  wires:
  Subsystem1/1(Out1) -> Mux2/2
  In1/1 -> Subsystem1/2(In2), Subsystem/2(In2)
  Subsystem/1(Out1) -> Mux2/1
  In2/1 -> Subsystem/1(In1)
  In3/1 -> Subsystem1/1(In1)
  Mux2/1 -> Out1/1

== system FKtest/Subsystem2 ==
  In1 : Inport
  In2 : Inport  Port=2
  In3 : Inport  Port=3
  Mux2 : Mux  Inputs=2
  Subsystem : Subsystem
  Subsystem1 : Subsystem
  Out1 : Outport
  wires:
  Subsystem1/1(Out1) -> Mux2/2
  In1/1 -> Subsystem1/2(In2), Subsystem/2(In2)
  Subsystem/1(Out1) -> Mux2/1
  In2/1 -> Subsystem/1(In1)
  In3/1 -> Subsystem1/1(In1)
  Mux2/1 -> Out1/1

== system FKtest/Subsystem3 ==
  In1 : Inport
  In2 : Inport  Port=2
  In3 : Inport  Port=3
  Mux2 : Mux  Inputs=2
  Subsystem : Subsystem
  Subsystem1 : Subsystem
  Out1 : Outport
  wires:
  Subsystem1/1(Out1) -> Mux2/2
  In1/1 -> Subsystem1/2(In2), Subsystem/2(In2)
  Subsystem/1(Out1) -> Mux2/1
  In2/1 -> Subsystem/1(In1)
  In3/1 -> Subsystem1/1(In1)
  Mux2/1 -> Out1/1

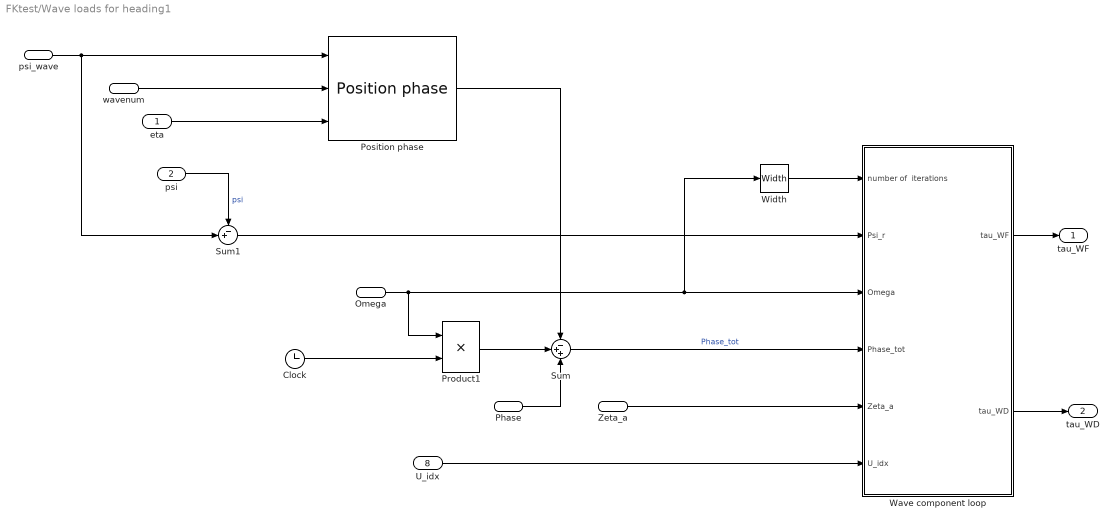
== system FKtest/Wave loads for heading1 ==
  eta : Inport
  psi : Inport  Port=2
  psi_wave : Inport  Port=3
  wavenum : Inport  Port=4
  Omega : Inport  Port=5
  Phase : Inport  Port=6
  Zeta_a : Inport  Port=7
  U_idx : Inport  Port=8
  Clock : Clock
      settings: Decimation=10
  Position phase : marine_gnc/Models/Environmental Loads/Utilities/Position phase  SystemSampleTime=-1
  Product1 : Product  Inputs=**  SaturateOnIntegerOverflow=on
  Sum : Sum  Inputs=-++  SaturateOnIntegerOverflow=on
  Sum1 : Sum  Inputs=-+|
  Wave component loop : Subsystem  TreatAsAtomicUnit=on
  Width : Width  DataType=int32
  tau_WF : Outport
  tau_WD : Outport  Port=2
  wires:
  Position phase/1 -> Sum/1
  Width/1 -> Wave component loop/1(number of  iterations)
  Sum/1 -> Wave component loop/4(Phase_tot)  "Phase_tot"
  Clock/1 -> Product1/2
  Product1/1 -> Sum/2
  Wave component loop/1(tau_WF) -> tau_WF/1
  eta/1 -> Position phase/3
  psi_wave/1 -> Position phase/1, Sum1/2
  wavenum/1 -> Position phase/2
  Omega/1 -> Product1/1, Wave component loop/3(Omega), Width/1
  Phase/1 -> Sum/3
  Zeta_a/1 -> Wave component loop/5(Zeta_a)
  Sum1/1 -> Wave component loop/2(Psi_r)
  Wave component loop/2(tau_WD) -> tau_WD/1
  U_idx/1 -> Wave component loop/6(U_idx)
  psi/1 -> Sum1/1  "psi"

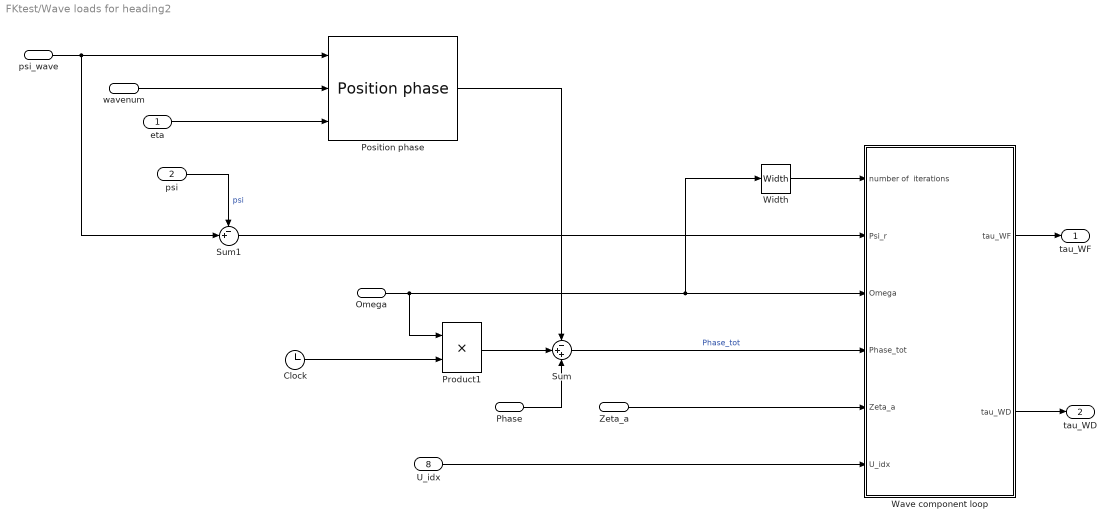
== system FKtest/Wave loads for heading2 ==
  eta : Inport
  psi : Inport  Port=2
  psi_wave : Inport  Port=3
  wavenum : Inport  Port=4
  Omega : Inport  Port=5
  Phase : Inport  Port=6
  Zeta_a : Inport  Port=7
  U_idx : Inport  Port=8
  Clock : Clock
      settings: Decimation=10
  Position phase : marine_gnc/Models/Environmental Loads/Utilities/Position phase  SystemSampleTime=-1
  Product1 : Product  Inputs=**  SaturateOnIntegerOverflow=on
  Sum : Sum  Inputs=-++  SaturateOnIntegerOverflow=on
  Sum1 : Sum  Inputs=-+|
  Wave component loop : Subsystem  TreatAsAtomicUnit=on
  Width : Width  DataType=int32
  tau_WF : Outport
  tau_WD : Outport  Port=2
  wires:
  Position phase/1 -> Sum/1
  Width/1 -> Wave component loop/1(number of  iterations)
  Sum/1 -> Wave component loop/4(Phase_tot)  "Phase_tot"
  Clock/1 -> Product1/2
  Product1/1 -> Sum/2
  Wave component loop/1(tau_WF) -> tau_WF/1
  eta/1 -> Position phase/3
  psi_wave/1 -> Position phase/1, Sum1/2
  wavenum/1 -> Position phase/2
  Omega/1 -> Product1/1, Wave component loop/3(Omega), Width/1
  Phase/1 -> Sum/3
  Zeta_a/1 -> Wave component loop/5(Zeta_a)
  Sum1/1 -> Wave component loop/2(Psi_r)
  Wave component loop/2(tau_WD) -> tau_WD/1
  U_idx/1 -> Wave component loop/6(U_idx)
  psi/1 -> Sum1/1  "psi"

== system FKtest/psi1 ==
  k : Inport  Orientation=down
  0 or 1 : Inport  Port=2
  Gain1 : Gain  Gain=20
  Gain2 : Gain  Gain=10
  Product : Product  RndMeth=Zero
  Sum7 : Sum  Inputs=-+|
  Sum8 : Sum  Inputs=++|
  const : Constant  Value=18
  psi : Outport
  wires:
  const/1 -> Sum7/2
  Sum7/1 -> Gain1/1
  Gain1/1 -> Product/1
  Product/1 -> Sum8/2
  Gain2/1 -> Sum8/1
  k/1 -> Sum7/1, Gain2/1
  Sum8/1 -> psi/1
  0 or 1/1 -> Product/2

== system FKtest/psi2 ==
  k : Inport  Orientation=down
  0 or 1 : Inport  Port=2
  Gain1 : Gain  Gain=20
  Gain2 : Gain  Gain=10
  Product : Product  RndMeth=Zero
  Sum7 : Sum  Inputs=-+|
  Sum8 : Sum  Inputs=++|
  const : Constant  Value=18
  psi : Outport
  wires:
  const/1 -> Sum7/2
  Sum7/1 -> Gain1/1
  Gain1/1 -> Product/1
  Product/1 -> Sum8/2
  Gain2/1 -> Sum8/1
  k/1 -> Sum7/1, Gain2/1
  Sum8/1 -> psi/1
  0 or 1/1 -> Product/2

== system FKtest/3 DOF wave drift/Output smoothing ==
  tau WD : Inport
  2nd order time constant {1..6} (6 alike) : marine_gnc/Utilities/Dynamics/2nd order time constant  SystemSampleTime=-1  T=RAO_smoothing_T
  Demux : Demux  Outputs=6
  Mux : Mux  Inputs=6
  "tau WD " : Outport
  wires:
  Demux/1 -> 2nd order time constant 1/1
  Demux/2 -> 2nd order time constant 2/1
  Demux/3 -> 2nd order time constant 3/1
  Demux/4 -> 2nd order time constant 4/1
  Demux/5 -> 2nd order time constant 5/1
  Demux/6 -> 2nd order time constant 6/1
  tau WD/1 -> Demux/1
  2nd order time constant 1/1 -> Mux/1
  2nd order time constant 2/1 -> Mux/2
  2nd order time constant 3/1 -> Mux/3
  2nd order time constant 4/1 -> Mux/4
  2nd order time constant 5/1 -> Mux/5
  2nd order time constant 6/1 -> Mux/6
  Mux/1 -> "tau WD "/1

== system FKtest/3 DOF wave drift/Wave component loop ==
  number of  iterations : Inport
  Psi_r : Inport  Port=2
  Omega : Inport  Port=3
  Zeta_a : Inport  Port=4
  vel : Inport  Port=5
  For Iterator : ForIterator  ResetStates=reset  IterationSource=external  IterationVariableDataType=double
  Memory2 : Memory  Orientation=left  X0=[0 0 0 0 0 0]'  InheritSampleTime=on
  Product4 : Product  Inputs=3  SaturateOnIntegerOverflow=on
  Selector2 : Selector  IndexOptions=Index vector (port)  Indices=[1 3]  OutputSizes=1
  Selector3 : Selector  IndexOptions=Index vector (port)  Indices=[1 3]  OutputSizes=1
  Selector4 : Selector  IndexOptions=Index vector (port)  Indices=[1 3]  OutputSizes=1
  Sum4 : Sum  Orientation=up  Inputs=++|  SaturateOnIntegerOverflow=on
  WD tables : Subsystem  mask(WD table lookup){RAO_Freq=WD_Freq, RAO_Dir=WD_Dir, RAO_Vel=WD_Vel, RAO_Amp=WD_Amp}
      mask prompts: RAO_Freq "Vector of frequencies (rad/s)"; RAO_Dir "Vector of directions (rad)"; RAO_Vel "Vector of velocities (m/s)"; RAO_Amp "6DOF Cell array with tables of Amplitudes"
      mask help: Perform 3D table lookup in 6DOF WD amplitudes, using the relative wave heading psi_r, wave frequency omega and vessel velocity vel as inputs.
  Tau WD : Outport
  wires:
  Selector3/1 -> WD tables/1(psi_r)  "psi_r"
  Selector2/1 -> WD tables/2(omega)  "omega"
  Product4/1 -> Sum4/1
  Memory2/1 -> Sum4/2
  Sum4/1 -> Memory2/1, Tau WD/1
  number of  iterations/1 -> For Iterator/1
  Omega/1 -> Selector2/1
  For Iterator/1 -> Selector4/2, Selector3/2, Selector2/2  "i=1:N"
  Psi_r/1 -> Selector3/1
  vel/1 -> WD tables/3(vel)
  WD tables/1(amp) -> Product4/1
  Zeta_a/1 -> Selector4/1
  Selector4/1 -> Product4/2, Product4/3  "zeta_a"

== system FKtest/3 DOF wave drift/Yaw quantizer ==
  psi LF : Inport
  psi wave : Inport  Port=2
  Backlash : Backlash  BacklashWidth=back
  Quantizer : Quantizer  QuantizationInterval=quant
  Quantizer flag : Constant  Value=quant_flag
  Sum : Sum  Inputs=|-+
  Switch : Switch  Threshold=0.5
  psi_r quantized : Outport
  wires:
  Quantizer/1 -> Switch/1
  Backlash/1 -> Quantizer/1
  psi LF/1 -> Backlash/1, Switch/3
  Sum/1 -> psi_r quantized/1
  psi wave/1 -> Sum/2
  Quantizer flag/1 -> Switch/2
  Switch/1 -> Sum/1

== system FKtest/Subsystem1/Subsystem ==
  In1 : Inport
  In2 : Inport  Port=2
  Integrator : Integrator
  Product4 : Product  Inputs=*/  RndMeth=Zero
  Out1 : Outport
  wires:
  Integrator/1 -> Product4/1
  In1/1 -> Integrator/1
  Product4/1 -> Out1/1
  In2/1 -> Product4/2

== system FKtest/Subsystem1/Subsystem1 ==
  In1 : Inport
  In2 : Inport  Port=2
  Integrator : Integrator
  Product4 : Product  Inputs=*/  RndMeth=Zero
  Out1 : Outport
  wires:
  Integrator/1 -> Product4/1
  In1/1 -> Integrator/1
  Product4/1 -> Out1/1
  In2/1 -> Product4/2
